simulink model "cic_filter_test_newnew_dec2_nonpoly_3"  (Simulink 7.4)
settings: Solver=ode45  StartTime=0.0  StopTime=50000  RelTol=1e-3
libraries: xbsIndex_r4 x203, simulink x3, xrbsComm_r4 x1, xps_library x1
(part 2 of 2)

== system cic_filter_test_newnew_dec2_nonpoly_3/CIC Filter/Integrator3 ==
  In1 : Inport  OutDataType=sfix(16)  OutScaling=2^0
  Accumulator : xbsIndex_r4/Accumulator  operation=Add  n_bits=output_bitwidth  overflow=Wrap  scale=1  rst=off  hasbypass=off  en=off  dbl_ovrd=off  use_behavioral_HDL=on  implementation=Fabric  block_type=accum
      settings: infoedit="Adder or subtractor-based accumulator.   Output type and binary point position match the input.<P><P>Hardware notes: When \"Reinitialize with Input 'b' on Reset\" is selected, the accumulator is forced to run at the system rate even if the input 'b' is running at a slower rate."  xl_area=[53 106 0 106 0 0 0]  block_version=VER_STRING_GOES_HERE
  Out1 : Outport  OutDataType=sfix(16)  OutScaling=2^0
  wires:
  Accumulator/1 -> Out1/1
  In1/1 -> Accumulator/1

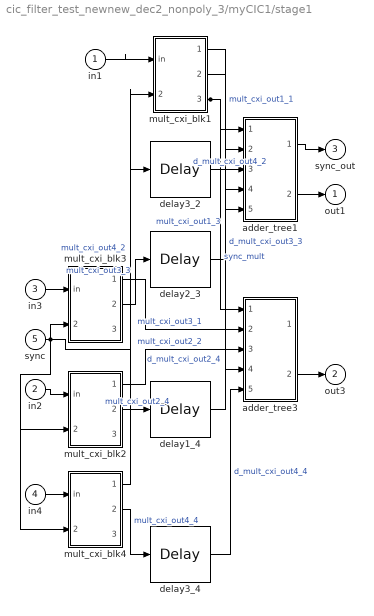
== system cic_filter_test_newnew_dec2_nonpoly_3/myCIC1/stage1 ==
  in1 : Inport
  in2 : Inport  Port=2
  in3 : Inport  Port=3
  in4 : Inport  Port=4
  sync : Inport  Port=5
  adder_tree1 : Subsystem
  adder_tree3 : Subsystem
  delay1_4 : xbsIndex_r4/Delay  en=off  latency=1  dbl_ovrd=off  reg_retiming=off  block_type=delay
      settings: block_version=11.4
  delay2_3 : xbsIndex_r4/Delay  en=off  latency=1  dbl_ovrd=off  reg_retiming=off  block_type=delay
      settings: block_version=11.4
  delay3_2 : xbsIndex_r4/Delay  en=off  latency=1  dbl_ovrd=off  reg_retiming=off  block_type=delay
      settings: block_version=11.4
  delay3_4 : xbsIndex_r4/Delay  en=off  latency=1  dbl_ovrd=off  reg_retiming=off  block_type=delay
      settings: block_version=11.4
  mult_cxi_blk1 : Subsystem
  mult_cxi_blk2 : Subsystem
  mult_cxi_blk3 : Subsystem
  mult_cxi_blk4 : Subsystem
  out1 : Outport
  out3 : Outport  Port=2
  sync_out : Outport  Port=3
  wires:
  sync/1 -> mult_cxi_blk4/2(sync), mult_cxi_blk2/2(sync), mult_cxi_blk1/2(sync), mult_cxi_blk3/2(sync)
  mult_cxi_blk1/3(sync_out) -> adder_tree3/1(sync), adder_tree1/1(sync)  "sync_mult"
  delay3_4/1 -> adder_tree3/5(din_4)  "d_mult_cxi_out4_4"
  mult_cxi_blk2/1(out1) -> adder_tree3/3(din_2)  "mult_cxi_out2_2"
  adder_tree1/2(dout) -> out1/1
  delay1_4/1 -> adder_tree1/5(din_4)  "d_mult_cxi_out2_4"
  delay3_2/1 -> adder_tree1/3(din_2)  "d_mult_cxi_out4_2"
  mult_cxi_blk4/2(out2) -> delay3_4/1  "mult_cxi_out4_4"
  mult_cxi_blk4/1(out1) -> delay3_2/1  "mult_cxi_out4_2"
  mult_cxi_blk3/2(out2) -> delay2_3/1  "mult_cxi_out3_3"
  mult_cxi_blk2/2(out2) -> delay1_4/1  "mult_cxi_out2_4"
  in3/1 -> mult_cxi_blk3/1(in)
  in1/1 -> mult_cxi_blk1/1(in)
  in2/1 -> mult_cxi_blk2/1(in)
  in4/1 -> mult_cxi_blk4/1(in)
  mult_cxi_blk1/1(out1) -> adder_tree1/2(din_1)  "mult_cxi_out1_1"
  delay2_3/1 -> adder_tree1/4(din_3)  "d_mult_cxi_out3_3"
  adder_tree1/1(sync_out) -> sync_out/1
  mult_cxi_blk3/1(out1) -> adder_tree3/2(din_1)  "mult_cxi_out3_1"
  mult_cxi_blk1/2(out2) -> adder_tree3/4(din_3)  "mult_cxi_out1_3"
  adder_tree3/2(dout) -> out3/1

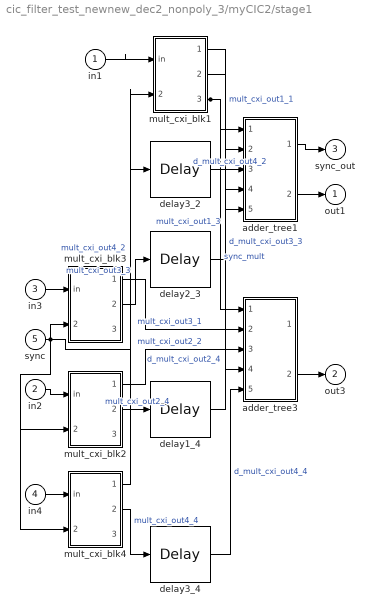
== system cic_filter_test_newnew_dec2_nonpoly_3/myCIC2/stage1 ==
  in1 : Inport
  in2 : Inport  Port=2
  in3 : Inport  Port=3
  in4 : Inport  Port=4
  sync : Inport  Port=5
  adder_tree1 : Subsystem
  adder_tree3 : Subsystem
  delay1_4 : xbsIndex_r4/Delay  en=off  latency=1  dbl_ovrd=off  reg_retiming=off  block_type=delay
      settings: block_version=11.4
  delay2_3 : xbsIndex_r4/Delay  en=off  latency=1  dbl_ovrd=off  reg_retiming=off  block_type=delay
      settings: block_version=11.4
  delay3_2 : xbsIndex_r4/Delay  en=off  latency=1  dbl_ovrd=off  reg_retiming=off  block_type=delay
      settings: block_version=11.4
  delay3_4 : xbsIndex_r4/Delay  en=off  latency=1  dbl_ovrd=off  reg_retiming=off  block_type=delay
      settings: block_version=11.4
  mult_cxi_blk1 : Subsystem
  mult_cxi_blk2 : Subsystem
  mult_cxi_blk3 : Subsystem
  mult_cxi_blk4 : Subsystem
  out1 : Outport
  out3 : Outport  Port=2
  sync_out : Outport  Port=3
  wires:
  sync/1 -> mult_cxi_blk4/2(sync), mult_cxi_blk2/2(sync), mult_cxi_blk1/2(sync), mult_cxi_blk3/2(sync)
  mult_cxi_blk1/3(sync_out) -> adder_tree3/1(sync), adder_tree1/1(sync)  "sync_mult"
  delay3_4/1 -> adder_tree3/5(din_4)  "d_mult_cxi_out4_4"
  mult_cxi_blk2/1(out1) -> adder_tree3/3(din_2)  "mult_cxi_out2_2"
  adder_tree1/2(dout) -> out1/1
  delay1_4/1 -> adder_tree1/5(din_4)  "d_mult_cxi_out2_4"
  delay3_2/1 -> adder_tree1/3(din_2)  "d_mult_cxi_out4_2"
  mult_cxi_blk4/2(out2) -> delay3_4/1  "mult_cxi_out4_4"
  mult_cxi_blk4/1(out1) -> delay3_2/1  "mult_cxi_out4_2"
  mult_cxi_blk3/2(out2) -> delay2_3/1  "mult_cxi_out3_3"
  mult_cxi_blk2/2(out2) -> delay1_4/1  "mult_cxi_out2_4"
  in3/1 -> mult_cxi_blk3/1(in)
  in1/1 -> mult_cxi_blk1/1(in)
  in2/1 -> mult_cxi_blk2/1(in)
  in4/1 -> mult_cxi_blk4/1(in)
  mult_cxi_blk1/1(out1) -> adder_tree1/2(din_1)  "mult_cxi_out1_1"
  delay2_3/1 -> adder_tree1/4(din_3)  "d_mult_cxi_out3_3"
  adder_tree1/1(sync_out) -> sync_out/1
  mult_cxi_blk3/1(out1) -> adder_tree3/2(din_1)  "mult_cxi_out3_1"
  mult_cxi_blk1/2(out2) -> adder_tree3/4(din_3)  "mult_cxi_out1_3"
  adder_tree3/2(dout) -> out3/1

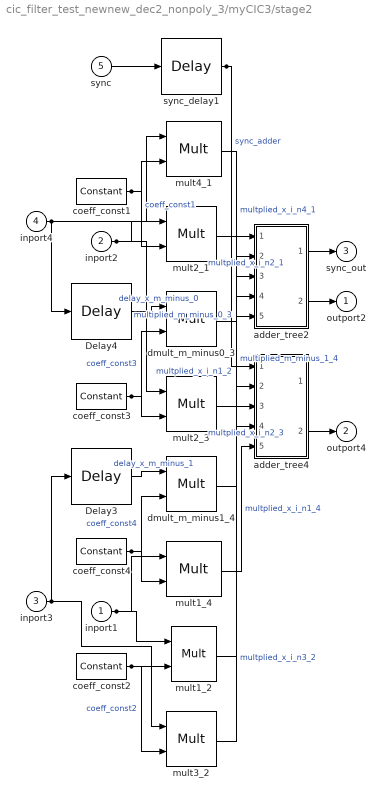
== system cic_filter_test_newnew_dec2_nonpoly_3/myCIC3/stage2 ==
  inport1 : Inport
  inport2 : Inport  Port=2
  inport3 : Inport  Port=3
  inport4 : Inport  Port=4
  sync : Inport  Port=5
  Delay3 : xbsIndex_r4/Delay  en=off  latency=1  dbl_ovrd=off  reg_retiming=off  block_type=delay
      settings: block_version=11.4
  Delay4 : xbsIndex_r4/Delay  en=off  latency=1  dbl_ovrd=off  reg_retiming=off  block_type=delay
      settings: block_version=11.4
  adder_tree2 : Subsystem
  adder_tree4 : Subsystem
  coeff_const1 : xbsIndex_r4/Constant  arith_type=Unsigned  const=1  n_bits=3  bin_pt=0  explicit_period=off  period=1  equ=P=C  opselect=C  inp2=PCIN>>17  opr=+  inp1=P  carry=CIN  dbl_ovrd=off  block_type=constant
      settings: block_version=11.4
  coeff_const2 : xbsIndex_r4/Constant  arith_type=Unsigned  const=3  n_bits=3  bin_pt=0  explicit_period=off  period=1  equ=P=C  opselect=C  inp2=PCIN>>17  opr=+  inp1=P  carry=CIN  dbl_ovrd=off  block_type=constant
      settings: block_version=11.4
  coeff_const3 : xbsIndex_r4/Constant  arith_type=Unsigned  const=3  n_bits=3  bin_pt=0  explicit_period=off  period=1  equ=P=C  opselect=C  inp2=PCIN>>17  opr=+  inp1=P  carry=CIN  dbl_ovrd=off  block_type=constant
      settings: block_version=11.4
  coeff_const4 : xbsIndex_r4/Constant  arith_type=Unsigned  const=1  n_bits=3  bin_pt=0  explicit_period=off  period=1  equ=P=C  opselect=C  inp2=PCIN>>17  opr=+  inp1=P  carry=CIN  dbl_ovrd=off  block_type=constant
      settings: block_version=11.4
  dmult_m_minus0_3 : xbsIndex_r4/Mult  precision=Full  arith_type="Signed  (2's comp)"  n_bits=16  bin_pt=14  quantization=Truncate  overflow=Wrap  en=off  latency=2  dbl_ovrd=off  use_behavioral_HDL=off  opt=Speed  use_embedded=on  optimum_pipeline=off  pipeline=on  use_rpm=on  placement_style=Triangular  block_type=mult
      settings: block_version=11.4
  dmult_m_minus1_4 : xbsIndex_r4/Mult  precision=Full  arith_type="Signed  (2's comp)"  n_bits=16  bin_pt=14  quantization=Truncate  overflow=Wrap  en=off  latency=2  dbl_ovrd=off  use_behavioral_HDL=off  opt=Speed  use_embedded=on  optimum_pipeline=off  pipeline=on  use_rpm=on  placement_style=Triangular  block_type=mult
      settings: block_version=11.4
  mult1_2 : xbsIndex_r4/Mult  precision=Full  arith_type="Signed  (2's comp)"  n_bits=16  bin_pt=14  quantization=Truncate  overflow=Wrap  en=off  latency=2  dbl_ovrd=off  use_behavioral_HDL=off  opt=Speed  use_embedded=on  optimum_pipeline=off  pipeline=on  use_rpm=on  placement_style=Triangular  block_type=mult
      settings: block_version=11.4
  mult1_4 : xbsIndex_r4/Mult  precision=Full  arith_type="Signed  (2's comp)"  n_bits=16  bin_pt=14  quantization=Truncate  overflow=Wrap  en=off  latency=2  dbl_ovrd=off  use_behavioral_HDL=off  opt=Speed  use_embedded=on  optimum_pipeline=off  pipeline=on  use_rpm=on  placement_style=Triangular  block_type=mult
      settings: block_version=11.4
  mult2_1 : xbsIndex_r4/Mult  precision=Full  arith_type="Signed  (2's comp)"  n_bits=16  bin_pt=14  quantization=Truncate  overflow=Wrap  en=off  latency=2  dbl_ovrd=off  use_behavioral_HDL=off  opt=Speed  use_embedded=on  optimum_pipeline=off  pipeline=on  use_rpm=on  placement_style=Triangular  block_type=mult
      settings: block_version=11.4
  mult2_3 : xbsIndex_r4/Mult  precision=Full  arith_type="Signed  (2's comp)"  n_bits=16  bin_pt=14  quantization=Truncate  overflow=Wrap  en=off  latency=2  dbl_ovrd=off  use_behavioral_HDL=off  opt=Speed  use_embedded=on  optimum_pipeline=off  pipeline=on  use_rpm=on  placement_style=Triangular  block_type=mult
      settings: block_version=11.4
  mult3_2 : xbsIndex_r4/Mult  precision=Full  arith_type="Signed  (2's comp)"  n_bits=16  bin_pt=14  quantization=Truncate  overflow=Wrap  en=off  latency=2  dbl_ovrd=off  use_behavioral_HDL=off  opt=Speed  use_embedded=on  optimum_pipeline=off  pipeline=on  use_rpm=on  placement_style=Triangular  block_type=mult
      settings: block_version=11.4
  mult4_1 : xbsIndex_r4/Mult  precision=Full  arith_type="Signed  (2's comp)"  n_bits=16  bin_pt=14  quantization=Truncate  overflow=Wrap  en=off  latency=2  dbl_ovrd=off  use_behavioral_HDL=off  opt=Speed  use_embedded=on  optimum_pipeline=off  pipeline=on  use_rpm=on  placement_style=Triangular  block_type=mult
      settings: block_version=11.4
  sync_delay1 : xbsIndex_r4/Delay  en=off  latency=2  dbl_ovrd=off  reg_retiming=off  block_type=delay
      settings: block_version=11.4
  outport2 : Outport
  outport4 : Outport  Port=2
  sync_out : Outport  Port=3
  wires:
  inport1/1 -> mult1_2/1, mult1_4/1
  coeff_const4/1 -> mult1_4/2, dmult_m_minus1_4/2  "coeff_const4"
  inport2/1 -> mult2_1/1, mult2_3/1
  coeff_const3/1 -> mult2_3/2, dmult_m_minus0_3/2  "coeff_const3"
  inport3/1 -> mult3_2/1, Delay3/1
  coeff_const2/1 -> mult1_2/2, mult3_2/2  "coeff_const2"
  inport4/1 -> Delay4/1, mult4_1/1
  coeff_const1/1 -> mult4_1/2, mult2_1/2  "coeff_const1"
  sync_delay1/1 -> adder_tree4/1(sync), adder_tree2/1(sync)  "sync_adder"
  mult1_4/1 -> adder_tree4/5(din_4)  "multplied_x_i_n1_4"
  mult3_2/1 -> adder_tree4/3(din_2)  "multplied_x_i_n3_2"
  adder_tree2/2(dout) -> outport2/1
  dmult_m_minus1_4/1 -> adder_tree2/5(din_4)  "multiplied_m_minus_1_4"
  mult1_2/1 -> adder_tree2/3(din_2)  "multplied_x_i_n1_2"
  sync/1 -> sync_delay1/1
  Delay4/1 -> dmult_m_minus0_3/1  "delay_x_m_minus_0"
  Delay3/1 -> dmult_m_minus1_4/1  "delay_x_m_minus_1"
  mult2_1/1 -> adder_tree2/2(din_1)  "multplied_x_i_n2_1"
  dmult_m_minus0_3/1 -> adder_tree2/4(din_3)  "multiplied_m_minus_0_3"
  adder_tree2/1(sync_out) -> sync_out/1
  mult4_1/1 -> adder_tree4/2(din_1)  "multplied_x_i_n4_1"
  mult2_3/1 -> adder_tree4/4(din_3)  "multplied_x_i_n2_3"
  adder_tree4/2(dout) -> outport4/1

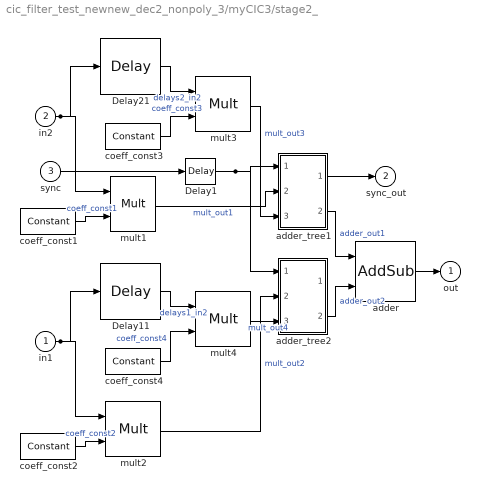
== system cic_filter_test_newnew_dec2_nonpoly_3/myCIC3/stage2_ ==
  in1 : Inport
  in2 : Inport  Port=2
  sync : Inport  Port=3
  Delay1 : xbsIndex_r4/Delay  en=off  latency=2  dbl_ovrd=off  reg_retiming=off  block_type=delay
      settings: block_version=11.4
  Delay11 : xbsIndex_r4/Delay  en=off  latency=1  dbl_ovrd=off  reg_retiming=off  block_type=delay
      settings: block_version=11.4
  Delay21 : xbsIndex_r4/Delay  en=off  latency=1  dbl_ovrd=off  reg_retiming=off  block_type=delay
      settings: block_version=11.4
  adder : xbsIndex_r4/AddSub  mode=Addition  use_carryin=off  use_carryout=off  en=off  latency=1  precision=Full  arith_type=Unsigned  n_bits=16  bin_pt=14  quantization=Truncate  overflow=Wrap  dbl_ovrd=off  use_behavioral_HDL=off  hw_selection=Fabric  pipelined=off  block_type=addsub
  adder_tree1 : Subsystem
  adder_tree2 : Subsystem
  coeff_const1 : xbsIndex_r4/Constant  arith_type=Unsigned  const=1  n_bits=3  bin_pt=0  explicit_period=off  period=1  equ=P=C  opselect=C  inp2=PCIN>>17  opr=+  inp1=P  carry=CIN  dbl_ovrd=off  block_type=constant
      settings: block_version=11.4
  coeff_const2 : xbsIndex_r4/Constant  arith_type=Unsigned  const=3  n_bits=3  bin_pt=0  explicit_period=off  period=1  equ=P=C  opselect=C  inp2=PCIN>>17  opr=+  inp1=P  carry=CIN  dbl_ovrd=off  block_type=constant
      settings: block_version=11.4
  coeff_const3 : xbsIndex_r4/Constant  arith_type=Unsigned  const=3  n_bits=3  bin_pt=0  explicit_period=off  period=1  equ=P=C  opselect=C  inp2=PCIN>>17  opr=+  inp1=P  carry=CIN  dbl_ovrd=off  block_type=constant
      settings: block_version=11.4
  coeff_const4 : xbsIndex_r4/Constant  arith_type=Unsigned  const=1  n_bits=3  bin_pt=0  explicit_period=off  period=1  equ=P=C  opselect=C  inp2=PCIN>>17  opr=+  inp1=P  carry=CIN  dbl_ovrd=off  block_type=constant
      settings: block_version=11.4
  mult{1..4} (4 alike) : xbsIndex_r4/Mult  precision=Full  arith_type="Signed  (2's comp)"  n_bits=16  bin_pt=14  quantization=Truncate  overflow=Wrap  en=off  latency=2  dbl_ovrd=off  use_behavioral_HDL=off  opt=Speed  use_embedded=on  optimum_pipeline=off  pipeline=on  use_rpm=on  placement_style=Triangular  block_type=mult
      settings: block_version=11.4
  out : Outport
  sync_out : Outport  Port=2
  wires:
  in2/1 -> mult1/1, Delay21/1
  in1/1 -> Delay11/1, mult2/1
  sync/1 -> Delay1/1
  adder_tree2/2(dout) -> adder/2  "adder_out2"
  mult2/1 -> adder_tree2/2(din_1)  "mult_out2"
  mult3/1 -> adder_tree1/3(din_2)  "mult_out3"
  coeff_const4/1 -> mult4/2  "coeff_const4"
  Delay21/1 -> mult3/1  "delays2_in2"
  coeff_const2/1 -> mult2/2  "coeff_const2"
  coeff_const1/1 -> mult1/2  "coeff_const1"
  coeff_const3/1 -> mult3/2  "coeff_const3"
  Delay11/1 -> mult4/1  "delays1_in2"
  mult1/1 -> adder_tree1/2(din_1)  "mult_out1"
  adder_tree1/1(sync_out) -> sync_out/1
  mult4/1 -> adder_tree2/3(din_2)  "mult_out4"
  adder_tree1/2(dout) -> adder/1  "adder_out1"
  adder/1 -> out/1
  Delay1/1 -> adder_tree1/1(sync), adder_tree2/1(sync)

== system cic_filter_test_newnew_dec2_nonpoly_3/npcic nonpoly/stage1 ==
  in : Inport
  sync : Inport  Port=2
  Down_sample0 : xbsIndex_r4/Down Sample  sample_ratio=2  sample_phase="Last Value of Frame  (most efficient)"  en=off  latency=1  dbl_ovrd=off  block_type=dsamp
      settings: block_version=11.4
  polynomial : Subsystem
  out : Outport
  sync_out : Outport  Port=2
  wires:
  polynomial/1(out) -> Down_sample0/1  "poly_out"
  polynomial/2(sync_out) -> sync_out/1
  in/1 -> polynomial/1(in)
  sync/1 -> polynomial/2(sync)
  Down_sample0/1 -> out/1

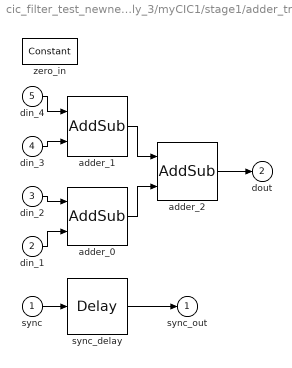
== system cic_filter_test_newnew_dec2_nonpoly_3/myCIC1/stage1/adder_tree1 ==
  sync : Inport
  din_1 : Inport  Port=2
  din_2 : Inport  Port=3
  din_3 : Inport  Port=4
  din_4 : Inport  Port=5
  adder_0 : xbsIndex_r4/AddSub  mode=Addition  use_carryin=off  use_carryout=off  en=off  latency=1  precision=Full  arith_type=Unsigned  n_bits=16  bin_pt=14  quantization="Round  (unbiased: +/- Inf)"  overflow=Saturate  dbl_ovrd=off  use_behavioral_HDL=on  hw_selection=Fabric  pipelined=off  block_type=addsub
  adder_1 : xbsIndex_r4/AddSub  mode=Addition  use_carryin=off  use_carryout=off  en=off  latency=1  precision=Full  arith_type=Unsigned  n_bits=16  bin_pt=14  quantization="Round  (unbiased: +/- Inf)"  overflow=Saturate  dbl_ovrd=off  use_behavioral_HDL=on  hw_selection=Fabric  pipelined=off  block_type=addsub
  adder_2 : xbsIndex_r4/AddSub  mode=Addition  use_carryin=off  use_carryout=off  en=off  latency=1  precision=Full  arith_type=Unsigned  n_bits=16  bin_pt=14  quantization="Round  (unbiased: +/- Inf)"  overflow=Saturate  dbl_ovrd=off  use_behavioral_HDL=on  hw_selection=Fabric  pipelined=off  block_type=addsub
  sync_delay : xbsIndex_r4/Delay  en=off  latency=2  dbl_ovrd=off  reg_retiming=off  block_type=delay
      settings: block_version=11.4
  zero_in : xbsIndex_r4/Constant  arith_type=Unsigned  const=0  n_bits=18  bin_pt=17  explicit_period=off  period=1  equ=P=C  opselect=C  inp2=PCIN>>17  opr=+  inp1=P  carry=CIN  dbl_ovrd=off  block_type=constant
      settings: block_version=11.4
  sync_out : Outport
  dout : Outport  Port=2
  wires:
  adder_0/1 -> adder_2/2
  din_4/1 -> adder_1/1
  din_1/1 -> adder_0/2
  sync_delay/1 -> sync_out/1
  sync/1 -> sync_delay/1
  din_2/1 -> adder_0/1
  din_3/1 -> adder_1/2
  adder_1/1 -> adder_2/1
  adder_2/1 -> dout/1

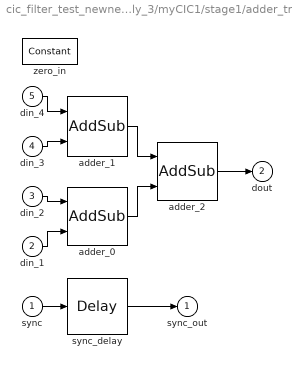
== system cic_filter_test_newnew_dec2_nonpoly_3/myCIC1/stage1/adder_tree3 ==
  sync : Inport
  din_1 : Inport  Port=2
  din_2 : Inport  Port=3
  din_3 : Inport  Port=4
  din_4 : Inport  Port=5
  adder_0 : xbsIndex_r4/AddSub  mode=Addition  use_carryin=off  use_carryout=off  en=off  latency=1  precision=Full  arith_type=Unsigned  n_bits=16  bin_pt=14  quantization="Round  (unbiased: +/- Inf)"  overflow=Saturate  dbl_ovrd=off  use_behavioral_HDL=on  hw_selection=Fabric  pipelined=off  block_type=addsub
  adder_1 : xbsIndex_r4/AddSub  mode=Addition  use_carryin=off  use_carryout=off  en=off  latency=1  precision=Full  arith_type=Unsigned  n_bits=16  bin_pt=14  quantization="Round  (unbiased: +/- Inf)"  overflow=Saturate  dbl_ovrd=off  use_behavioral_HDL=on  hw_selection=Fabric  pipelined=off  block_type=addsub
  adder_2 : xbsIndex_r4/AddSub  mode=Addition  use_carryin=off  use_carryout=off  en=off  latency=1  precision=Full  arith_type=Unsigned  n_bits=16  bin_pt=14  quantization="Round  (unbiased: +/- Inf)"  overflow=Saturate  dbl_ovrd=off  use_behavioral_HDL=on  hw_selection=Fabric  pipelined=off  block_type=addsub
  sync_delay : xbsIndex_r4/Delay  en=off  latency=2  dbl_ovrd=off  reg_retiming=off  block_type=delay
      settings: block_version=11.4
  zero_in : xbsIndex_r4/Constant  arith_type=Unsigned  const=0  n_bits=18  bin_pt=17  explicit_period=off  period=1  equ=P=C  opselect=C  inp2=PCIN>>17  opr=+  inp1=P  carry=CIN  dbl_ovrd=off  block_type=constant
      settings: block_version=11.4
  sync_out : Outport
  dout : Outport  Port=2
  wires:
  adder_0/1 -> adder_2/2
  din_4/1 -> adder_1/1
  din_1/1 -> adder_0/2
  sync_delay/1 -> sync_out/1
  sync/1 -> sync_delay/1
  din_2/1 -> adder_0/1
  din_3/1 -> adder_1/2
  adder_1/1 -> adder_2/1
  adder_2/1 -> dout/1

== system cic_filter_test_newnew_dec2_nonpoly_3/myCIC1/stage1/mult_cxi_blk1 ==
  in : Inport
  sync : Inport  Port=2
  adder_tree2 : Subsystem
  delay1 : xbsIndex_r4/Delay  en=off  latency=1  dbl_ovrd=off  reg_retiming=off  block_type=delay
      settings: block_version=11.4
  shift2 : xbsIndex_r4/Shift  shift_dir=Left  shift_bits=1  en=off  latency=0  precision=Full  arith_type="Signed  (2's comp)"  n_bits=16  bin_pt=14  quantization=Truncate  overflow=Wrap  dbl_ovrd=off  block_type=shift
  sync_delay : xbsIndex_r4/Delay  en=off  latency=1  dbl_ovrd=off  reg_retiming=off  block_type=delay
      settings: block_version=11.4
  out1 : Outport
  out2 : Outport  Port=2
  sync_out : Outport  Port=3
  wires:
  in/1 -> delay1/1, adder_tree2/1(sync), shift2/1, adder_tree2/2(din_1)  "adder_trees_out1"
  sync/1 -> sync_delay/1
  delay1/1 -> out1/1  "out1"
  shift2/1 -> adder_tree2/3(din_2)  "shift_out2"
  adder_tree2/2(dout) -> out2/1  "out2"
  sync_delay/1 -> sync_out/1

== system cic_filter_test_newnew_dec2_nonpoly_3/myCIC1/stage1/mult_cxi_blk2 ==
  in : Inport
  sync : Inport  Port=2
  adder_tree1 : Subsystem
  delay2 : xbsIndex_r4/Delay  en=off  latency=1  dbl_ovrd=off  reg_retiming=off  block_type=delay
      settings: block_version=11.4
  shift2 : xbsIndex_r4/Shift  shift_dir=Left  shift_bits=1  en=off  latency=0  precision=Full  arith_type="Signed  (2's comp)"  n_bits=16  bin_pt=14  quantization=Truncate  overflow=Wrap  dbl_ovrd=off  block_type=shift
  sync_delay : xbsIndex_r4/Delay  en=off  latency=1  dbl_ovrd=off  reg_retiming=off  block_type=delay
      settings: block_version=11.4
  out1 : Outport
  out2 : Outport  Port=2
  sync_out : Outport  Port=3
  wires:
  in/1 -> delay2/1, adder_tree1/1(sync), shift2/1, adder_tree1/2(din_1)  "adder_trees_out2"
  sync/1 -> sync_delay/1
  adder_tree1/2(dout) -> out1/1  "out1"
  shift2/1 -> adder_tree1/3(din_2)  "shift_out2"
  delay2/1 -> out2/1  "out2"
  sync_delay/1 -> sync_out/1

== system cic_filter_test_newnew_dec2_nonpoly_3/myCIC1/stage1/mult_cxi_blk3 ==
  in : Inport
  sync : Inport  Port=2
  adder_tree2 : Subsystem
  delay1 : xbsIndex_r4/Delay  en=off  latency=1  dbl_ovrd=off  reg_retiming=off  block_type=delay
      settings: block_version=11.4
  shift2 : xbsIndex_r4/Shift  shift_dir=Left  shift_bits=1  en=off  latency=0  precision=Full  arith_type="Signed  (2's comp)"  n_bits=16  bin_pt=14  quantization=Truncate  overflow=Wrap  dbl_ovrd=off  block_type=shift
  sync_delay : xbsIndex_r4/Delay  en=off  latency=1  dbl_ovrd=off  reg_retiming=off  block_type=delay
      settings: block_version=11.4
  out1 : Outport
  out2 : Outport  Port=2
  sync_out : Outport  Port=3
  wires:
  in/1 -> delay1/1, adder_tree2/1(sync), shift2/1, adder_tree2/2(din_1)  "adder_trees_out1"
  sync/1 -> sync_delay/1
  delay1/1 -> out1/1  "out1"
  shift2/1 -> adder_tree2/3(din_2)  "shift_out2"
  adder_tree2/2(dout) -> out2/1  "out2"
  sync_delay/1 -> sync_out/1

== system cic_filter_test_newnew_dec2_nonpoly_3/myCIC1/stage1/mult_cxi_blk4 ==
  in : Inport
  sync : Inport  Port=2
  adder_tree1 : Subsystem
  delay2 : xbsIndex_r4/Delay  en=off  latency=1  dbl_ovrd=off  reg_retiming=off  block_type=delay
      settings: block_version=11.4
  shift2 : xbsIndex_r4/Shift  shift_dir=Left  shift_bits=1  en=off  latency=0  precision=Full  arith_type="Signed  (2's comp)"  n_bits=16  bin_pt=14  quantization=Truncate  overflow=Wrap  dbl_ovrd=off  block_type=shift
  sync_delay : xbsIndex_r4/Delay  en=off  latency=1  dbl_ovrd=off  reg_retiming=off  block_type=delay
      settings: block_version=11.4
  out1 : Outport
  out2 : Outport  Port=2
  sync_out : Outport  Port=3
  wires:
  in/1 -> delay2/1, adder_tree1/1(sync), shift2/1, adder_tree1/2(din_1)  "adder_trees_out2"
  sync/1 -> sync_delay/1
  adder_tree1/2(dout) -> out1/1  "out1"
  shift2/1 -> adder_tree1/3(din_2)  "shift_out2"
  delay2/1 -> out2/1  "out2"
  sync_delay/1 -> sync_out/1

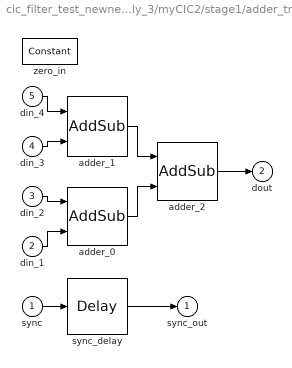
== system cic_filter_test_newnew_dec2_nonpoly_3/myCIC2/stage1/adder_tree1 ==
  sync : Inport
  din_1 : Inport  Port=2
  din_2 : Inport  Port=3
  din_3 : Inport  Port=4
  din_4 : Inport  Port=5
  adder_0 : xbsIndex_r4/AddSub  mode=Addition  use_carryin=off  use_carryout=off  en=off  latency=1  precision=Full  arith_type=Unsigned  n_bits=16  bin_pt=14  quantization="Round  (unbiased: +/- Inf)"  overflow=Saturate  dbl_ovrd=off  use_behavioral_HDL=on  hw_selection=Fabric  pipelined=off  block_type=addsub
  adder_1 : xbsIndex_r4/AddSub  mode=Addition  use_carryin=off  use_carryout=off  en=off  latency=1  precision=Full  arith_type=Unsigned  n_bits=16  bin_pt=14  quantization="Round  (unbiased: +/- Inf)"  overflow=Saturate  dbl_ovrd=off  use_behavioral_HDL=on  hw_selection=Fabric  pipelined=off  block_type=addsub
  adder_2 : xbsIndex_r4/AddSub  mode=Addition  use_carryin=off  use_carryout=off  en=off  latency=1  precision=Full  arith_type=Unsigned  n_bits=16  bin_pt=14  quantization="Round  (unbiased: +/- Inf)"  overflow=Saturate  dbl_ovrd=off  use_behavioral_HDL=on  hw_selection=Fabric  pipelined=off  block_type=addsub
  sync_delay : xbsIndex_r4/Delay  en=off  latency=2  dbl_ovrd=off  reg_retiming=off  block_type=delay
      settings: block_version=11.4
  zero_in : xbsIndex_r4/Constant  arith_type=Unsigned  const=0  n_bits=18  bin_pt=17  explicit_period=off  period=1  equ=P=C  opselect=C  inp2=PCIN>>17  opr=+  inp1=P  carry=CIN  dbl_ovrd=off  block_type=constant
      settings: block_version=11.4
  sync_out : Outport
  dout : Outport  Port=2
  wires:
  adder_0/1 -> adder_2/2
  din_4/1 -> adder_1/1
  din_1/1 -> adder_0/2
  sync_delay/1 -> sync_out/1
  sync/1 -> sync_delay/1
  din_2/1 -> adder_0/1
  din_3/1 -> adder_1/2
  adder_1/1 -> adder_2/1
  adder_2/1 -> dout/1

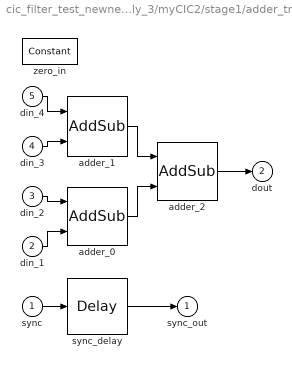
== system cic_filter_test_newnew_dec2_nonpoly_3/myCIC2/stage1/adder_tree3 ==
  sync : Inport
  din_1 : Inport  Port=2
  din_2 : Inport  Port=3
  din_3 : Inport  Port=4
  din_4 : Inport  Port=5
  adder_0 : xbsIndex_r4/AddSub  mode=Addition  use_carryin=off  use_carryout=off  en=off  latency=1  precision=Full  arith_type=Unsigned  n_bits=16  bin_pt=14  quantization="Round  (unbiased: +/- Inf)"  overflow=Saturate  dbl_ovrd=off  use_behavioral_HDL=on  hw_selection=Fabric  pipelined=off  block_type=addsub
  adder_1 : xbsIndex_r4/AddSub  mode=Addition  use_carryin=off  use_carryout=off  en=off  latency=1  precision=Full  arith_type=Unsigned  n_bits=16  bin_pt=14  quantization="Round  (unbiased: +/- Inf)"  overflow=Saturate  dbl_ovrd=off  use_behavioral_HDL=on  hw_selection=Fabric  pipelined=off  block_type=addsub
  adder_2 : xbsIndex_r4/AddSub  mode=Addition  use_carryin=off  use_carryout=off  en=off  latency=1  precision=Full  arith_type=Unsigned  n_bits=16  bin_pt=14  quantization="Round  (unbiased: +/- Inf)"  overflow=Saturate  dbl_ovrd=off  use_behavioral_HDL=on  hw_selection=Fabric  pipelined=off  block_type=addsub
  sync_delay : xbsIndex_r4/Delay  en=off  latency=2  dbl_ovrd=off  reg_retiming=off  block_type=delay
      settings: block_version=11.4
  zero_in : xbsIndex_r4/Constant  arith_type=Unsigned  const=0  n_bits=18  bin_pt=17  explicit_period=off  period=1  equ=P=C  opselect=C  inp2=PCIN>>17  opr=+  inp1=P  carry=CIN  dbl_ovrd=off  block_type=constant
      settings: block_version=11.4
  sync_out : Outport
  dout : Outport  Port=2
  wires:
  adder_0/1 -> adder_2/2
  din_4/1 -> adder_1/1
  din_1/1 -> adder_0/2
  sync_delay/1 -> sync_out/1
  sync/1 -> sync_delay/1
  din_2/1 -> adder_0/1
  din_3/1 -> adder_1/2
  adder_1/1 -> adder_2/1
  adder_2/1 -> dout/1

== system cic_filter_test_newnew_dec2_nonpoly_3/myCIC2/stage1/mult_cxi_blk1 ==
  in : Inport
  sync : Inport  Port=2
  adder_tree2 : Subsystem
  delay1 : xbsIndex_r4/Delay  en=off  latency=1  dbl_ovrd=off  reg_retiming=off  block_type=delay
      settings: block_version=11.4
  shift2 : xbsIndex_r4/Shift  shift_dir=Left  shift_bits=1  en=off  latency=0  precision=Full  arith_type="Signed  (2's comp)"  n_bits=16  bin_pt=14  quantization=Truncate  overflow=Wrap  dbl_ovrd=off  block_type=shift
  sync_delay : xbsIndex_r4/Delay  en=off  latency=1  dbl_ovrd=off  reg_retiming=off  block_type=delay
      settings: block_version=11.4
  out1 : Outport
  out2 : Outport  Port=2
  sync_out : Outport  Port=3
  wires:
  in/1 -> delay1/1, adder_tree2/1(sync), shift2/1, adder_tree2/2(din_1)  "adder_trees_out1"
  sync/1 -> sync_delay/1
  delay1/1 -> out1/1  "out1"
  shift2/1 -> adder_tree2/3(din_2)  "shift_out2"
  adder_tree2/2(dout) -> out2/1  "out2"
  sync_delay/1 -> sync_out/1

== system cic_filter_test_newnew_dec2_nonpoly_3/myCIC2/stage1/mult_cxi_blk2 ==
  in : Inport
  sync : Inport  Port=2
  adder_tree1 : Subsystem
  delay2 : xbsIndex_r4/Delay  en=off  latency=1  dbl_ovrd=off  reg_retiming=off  block_type=delay
      settings: block_version=11.4
  shift2 : xbsIndex_r4/Shift  shift_dir=Left  shift_bits=1  en=off  latency=0  precision=Full  arith_type="Signed  (2's comp)"  n_bits=16  bin_pt=14  quantization=Truncate  overflow=Wrap  dbl_ovrd=off  block_type=shift
  sync_delay : xbsIndex_r4/Delay  en=off  latency=1  dbl_ovrd=off  reg_retiming=off  block_type=delay
      settings: block_version=11.4
  out1 : Outport
  out2 : Outport  Port=2
  sync_out : Outport  Port=3
  wires:
  in/1 -> delay2/1, adder_tree1/1(sync), shift2/1, adder_tree1/2(din_1)  "adder_trees_out2"
  sync/1 -> sync_delay/1
  adder_tree1/2(dout) -> out1/1  "out1"
  shift2/1 -> adder_tree1/3(din_2)  "shift_out2"
  delay2/1 -> out2/1  "out2"
  sync_delay/1 -> sync_out/1

== system cic_filter_test_newnew_dec2_nonpoly_3/myCIC2/stage1/mult_cxi_blk3 ==
  in : Inport
  sync : Inport  Port=2
  adder_tree2 : Subsystem
  delay1 : xbsIndex_r4/Delay  en=off  latency=1  dbl_ovrd=off  reg_retiming=off  block_type=delay
      settings: block_version=11.4
  shift2 : xbsIndex_r4/Shift  shift_dir=Left  shift_bits=1  en=off  latency=0  precision=Full  arith_type="Signed  (2's comp)"  n_bits=16  bin_pt=14  quantization=Truncate  overflow=Wrap  dbl_ovrd=off  block_type=shift
  sync_delay : xbsIndex_r4/Delay  en=off  latency=1  dbl_ovrd=off  reg_retiming=off  block_type=delay
      settings: block_version=11.4
  out1 : Outport
  out2 : Outport  Port=2
  sync_out : Outport  Port=3
  wires:
  in/1 -> delay1/1, adder_tree2/1(sync), shift2/1, adder_tree2/2(din_1)  "adder_trees_out1"
  sync/1 -> sync_delay/1
  delay1/1 -> out1/1  "out1"
  shift2/1 -> adder_tree2/3(din_2)  "shift_out2"
  adder_tree2/2(dout) -> out2/1  "out2"
  sync_delay/1 -> sync_out/1

== system cic_filter_test_newnew_dec2_nonpoly_3/myCIC2/stage1/mult_cxi_blk4 ==
  in : Inport
  sync : Inport  Port=2
  adder_tree1 : Subsystem
  delay2 : xbsIndex_r4/Delay  en=off  latency=1  dbl_ovrd=off  reg_retiming=off  block_type=delay
      settings: block_version=11.4
  shift2 : xbsIndex_r4/Shift  shift_dir=Left  shift_bits=1  en=off  latency=0  precision=Full  arith_type="Signed  (2's comp)"  n_bits=16  bin_pt=14  quantization=Truncate  overflow=Wrap  dbl_ovrd=off  block_type=shift
  sync_delay : xbsIndex_r4/Delay  en=off  latency=1  dbl_ovrd=off  reg_retiming=off  block_type=delay
      settings: block_version=11.4
  out1 : Outport
  out2 : Outport  Port=2
  sync_out : Outport  Port=3
  wires:
  in/1 -> delay2/1, adder_tree1/1(sync), shift2/1, adder_tree1/2(din_1)  "adder_trees_out2"
  sync/1 -> sync_delay/1
  adder_tree1/2(dout) -> out1/1  "out1"
  shift2/1 -> adder_tree1/3(din_2)  "shift_out2"
  delay2/1 -> out2/1  "out2"
  sync_delay/1 -> sync_out/1

== system cic_filter_test_newnew_dec2_nonpoly_3/myCIC3/stage2/adder_tree2 ==
  sync : Inport
  din_1 : Inport  Port=2
  din_2 : Inport  Port=3
  din_3 : Inport  Port=4
  din_4 : Inport  Port=5
  adder_0 : xbsIndex_r4/AddSub  mode=Addition  use_carryin=off  use_carryout=off  en=off  latency=1  precision=Full  arith_type=Unsigned  n_bits=16  bin_pt=14  quantization="Round  (unbiased: +/- Inf)"  overflow=Saturate  dbl_ovrd=off  use_behavioral_HDL=on  hw_selection=Fabric  pipelined=off  block_type=addsub
  adder_1 : xbsIndex_r4/AddSub  mode=Addition  use_carryin=off  use_carryout=off  en=off  latency=1  precision=Full  arith_type=Unsigned  n_bits=16  bin_pt=14  quantization="Round  (unbiased: +/- Inf)"  overflow=Saturate  dbl_ovrd=off  use_behavioral_HDL=on  hw_selection=Fabric  pipelined=off  block_type=addsub
  adder_2 : xbsIndex_r4/AddSub  mode=Addition  use_carryin=off  use_carryout=off  en=off  latency=1  precision=Full  arith_type=Unsigned  n_bits=16  bin_pt=14  quantization="Round  (unbiased: +/- Inf)"  overflow=Saturate  dbl_ovrd=off  use_behavioral_HDL=on  hw_selection=Fabric  pipelined=off  block_type=addsub
  sync_delay : xbsIndex_r4/Delay  en=off  latency=2  dbl_ovrd=off  reg_retiming=off  block_type=delay
      settings: block_version=11.4
  zero_in : xbsIndex_r4/Constant  arith_type=Unsigned  const=0  n_bits=18  bin_pt=17  explicit_period=off  period=1  equ=P=C  opselect=C  inp2=PCIN>>17  opr=+  inp1=P  carry=CIN  dbl_ovrd=off  block_type=constant
      settings: block_version=11.4
  sync_out : Outport
  dout : Outport  Port=2
  wires:
  adder_0/1 -> adder_2/2
  din_4/1 -> adder_1/1
  din_1/1 -> adder_0/2
  sync_delay/1 -> sync_out/1
  sync/1 -> sync_delay/1
  din_2/1 -> adder_0/1
  din_3/1 -> adder_1/2
  adder_1/1 -> adder_2/1
  adder_2/1 -> dout/1

== system cic_filter_test_newnew_dec2_nonpoly_3/myCIC3/stage2/adder_tree4 ==
  sync : Inport
  din_1 : Inport  Port=2
  din_2 : Inport  Port=3
  din_3 : Inport  Port=4
  din_4 : Inport  Port=5
  adder_0 : xbsIndex_r4/AddSub  mode=Addition  use_carryin=off  use_carryout=off  en=off  latency=1  precision=Full  arith_type=Unsigned  n_bits=16  bin_pt=14  quantization="Round  (unbiased: +/- Inf)"  overflow=Saturate  dbl_ovrd=off  use_behavioral_HDL=on  hw_selection=Fabric  pipelined=off  block_type=addsub
  adder_1 : xbsIndex_r4/AddSub  mode=Addition  use_carryin=off  use_carryout=off  en=off  latency=1  precision=Full  arith_type=Unsigned  n_bits=16  bin_pt=14  quantization="Round  (unbiased: +/- Inf)"  overflow=Saturate  dbl_ovrd=off  use_behavioral_HDL=on  hw_selection=Fabric  pipelined=off  block_type=addsub
  adder_2 : xbsIndex_r4/AddSub  mode=Addition  use_carryin=off  use_carryout=off  en=off  latency=1  precision=Full  arith_type=Unsigned  n_bits=16  bin_pt=14  quantization="Round  (unbiased: +/- Inf)"  overflow=Saturate  dbl_ovrd=off  use_behavioral_HDL=on  hw_selection=Fabric  pipelined=off  block_type=addsub
  sync_delay : xbsIndex_r4/Delay  en=off  latency=2  dbl_ovrd=off  reg_retiming=off  block_type=delay
      settings: block_version=11.4
  zero_in : xbsIndex_r4/Constant  arith_type=Unsigned  const=0  n_bits=18  bin_pt=17  explicit_period=off  period=1  equ=P=C  opselect=C  inp2=PCIN>>17  opr=+  inp1=P  carry=CIN  dbl_ovrd=off  block_type=constant
      settings: block_version=11.4
  sync_out : Outport
  dout : Outport  Port=2
  wires:
  adder_0/1 -> adder_2/2
  din_4/1 -> adder_1/1
  din_1/1 -> adder_0/2
  sync_delay/1 -> sync_out/1
  sync/1 -> sync_delay/1
  din_2/1 -> adder_0/1
  din_3/1 -> adder_1/2
  adder_1/1 -> adder_2/1
  adder_2/1 -> dout/1

== system cic_filter_test_newnew_dec2_nonpoly_3/myCIC3/stage2_/adder_tree1 ==
  sync : Inport
  din_1 : Inport  Port=2
  din_2 : Inport  Port=3
  adder_0 : xbsIndex_r4/AddSub  mode=Addition  use_carryin=off  use_carryout=off  en=off  latency=1  precision=Full  arith_type=Unsigned  n_bits=16  bin_pt=14  quantization="Round  (unbiased: +/- Inf)"  overflow=Saturate  dbl_ovrd=off  use_behavioral_HDL=on  hw_selection=Fabric  pipelined=off  block_type=addsub
  sync_delay : xbsIndex_r4/Delay  en=off  latency=1  dbl_ovrd=off  reg_retiming=off  block_type=delay
      settings: block_version=11.4
  zero_in : xbsIndex_r4/Constant  arith_type=Unsigned  const=0  n_bits=18  bin_pt=17  explicit_period=off  period=1  equ=P=C  opselect=C  inp2=PCIN>>17  opr=+  inp1=P  carry=CIN  dbl_ovrd=off  block_type=constant
      settings: block_version=11.4
  sync_out : Outport
  dout : Outport  Port=2
  wires:
  din_1/1 -> adder_0/2
  sync_delay/1 -> sync_out/1
  sync/1 -> sync_delay/1
  din_2/1 -> adder_0/1
  adder_0/1 -> dout/1

== system cic_filter_test_newnew_dec2_nonpoly_3/myCIC3/stage2_/adder_tree2 ==
  sync : Inport
  din_1 : Inport  Port=2
  din_2 : Inport  Port=3
  adder_0 : xbsIndex_r4/AddSub  mode=Addition  use_carryin=off  use_carryout=off  en=off  latency=1  precision=Full  arith_type=Unsigned  n_bits=16  bin_pt=14  quantization="Round  (unbiased: +/- Inf)"  overflow=Saturate  dbl_ovrd=off  use_behavioral_HDL=on  hw_selection=Fabric  pipelined=off  block_type=addsub
  sync_delay : xbsIndex_r4/Delay  en=off  latency=1  dbl_ovrd=off  reg_retiming=off  block_type=delay
      settings: block_version=11.4
  zero_in : xbsIndex_r4/Constant  arith_type=Unsigned  const=0  n_bits=18  bin_pt=17  explicit_period=off  period=1  equ=P=C  opselect=C  inp2=PCIN>>17  opr=+  inp1=P  carry=CIN  dbl_ovrd=off  block_type=constant
      settings: block_version=11.4
  sync_out : Outport
  dout : Outport  Port=2
  wires:
  din_1/1 -> adder_0/2
  sync_delay/1 -> sync_out/1
  sync/1 -> sync_delay/1
  din_2/1 -> adder_0/1
  adder_0/1 -> dout/1

== system cic_filter_test_newnew_dec2_nonpoly_3/npcic nonpoly/stage1/polynomial ==
  in : Inport
  sync : Inport  Port=2
  adder_blk1 : xbsIndex_r4/AddSub  mode=Addition  use_carryin=off  use_carryout=off  en=off  latency=1  precision=Full  arith_type=Unsigned  n_bits=16  bin_pt=14  quantization=Truncate  overflow=Wrap  dbl_ovrd=off  use_behavioral_HDL=off  hw_selection=Fabric  pipelined=off  block_type=addsub
  adder_blk2 : xbsIndex_r4/AddSub  mode=Addition  use_carryin=off  use_carryout=off  en=off  latency=1  precision=Full  arith_type=Unsigned  n_bits=16  bin_pt=14  quantization=Truncate  overflow=Wrap  dbl_ovrd=off  use_behavioral_HDL=off  hw_selection=Fabric  pipelined=off  block_type=addsub
  adder_blk3 : xbsIndex_r4/AddSub  mode=Addition  use_carryin=off  use_carryout=off  en=off  latency=1  precision=Full  arith_type=Unsigned  n_bits=16  bin_pt=14  quantization=Truncate  overflow=Wrap  dbl_ovrd=off  use_behavioral_HDL=off  hw_selection=Fabric  pipelined=off  block_type=addsub
  delay0 : xbsIndex_r4/Delay  en=off  latency=1  dbl_ovrd=off  reg_retiming=off  block_type=delay
      settings: block_version=11.4
  shift_mult_array : Subsystem
  sync_delay1 : xbsIndex_r4/Delay  en=off  latency=1  dbl_ovrd=off  reg_retiming=off  block_type=delay
      settings: block_version=11.4
  out : Outport
  sync_out : Outport  Port=2
  wires:
  shift_mult_array/5(sync_out) -> sync_delay1/1  "sync_mult"
  adder_blk2/1 -> adder_blk3/1  "adder_ins3"
  shift_mult_array/3(out3) -> adder_blk2/2  "mult_out3"
  delay0/1 -> adder_blk1/1  "adder_ins1"
  shift_mult_array/1(out1) -> delay0/1  "mult_out1"
  sync/1 -> shift_mult_array/2(sync)
  in/1 -> shift_mult_array/1(in)
  shift_mult_array/2(out2) -> adder_blk1/2  "mult_out2"
  adder_blk1/1 -> adder_blk2/1  "adder_ins2"
  shift_mult_array/4(out4) -> adder_blk3/2  "mult_out4"
  adder_blk3/1 -> out/1  "adder_ins4"
  sync_delay1/1 -> sync_out/1

== system cic_filter_test_newnew_dec2_nonpoly_3/myCIC1/stage1/mult_cxi_blk1/adder_tree2 ==
  sync : Inport
  din_1 : Inport  Port=2
  din_2 : Inport  Port=3
  adder_0 : xbsIndex_r4/AddSub  mode=Addition  use_carryin=off  use_carryout=off  en=off  latency=1  precision=Full  arith_type=Unsigned  n_bits=16  bin_pt=14  quantization="Round  (unbiased: +/- Inf)"  overflow=Saturate  dbl_ovrd=off  use_behavioral_HDL=on  hw_selection=Fabric  pipelined=off  block_type=addsub
  sync_delay : xbsIndex_r4/Delay  en=off  latency=1  dbl_ovrd=off  reg_retiming=off  block_type=delay
      settings: block_version=11.4
  zero_in : xbsIndex_r4/Constant  arith_type=Unsigned  const=0  n_bits=18  bin_pt=17  explicit_period=off  period=1  equ=P=C  opselect=C  inp2=PCIN>>17  opr=+  inp1=P  carry=CIN  dbl_ovrd=off  block_type=constant
      settings: block_version=11.4
  sync_out : Outport
  dout : Outport  Port=2
  wires:
  din_1/1 -> adder_0/2
  sync_delay/1 -> sync_out/1
  sync/1 -> sync_delay/1
  din_2/1 -> adder_0/1
  adder_0/1 -> dout/1

== system cic_filter_test_newnew_dec2_nonpoly_3/myCIC1/stage1/mult_cxi_blk2/adder_tree1 ==
  sync : Inport
  din_1 : Inport  Port=2
  din_2 : Inport  Port=3
  adder_0 : xbsIndex_r4/AddSub  mode=Addition  use_carryin=off  use_carryout=off  en=off  latency=1  precision=Full  arith_type=Unsigned  n_bits=16  bin_pt=14  quantization="Round  (unbiased: +/- Inf)"  overflow=Saturate  dbl_ovrd=off  use_behavioral_HDL=on  hw_selection=Fabric  pipelined=off  block_type=addsub
  sync_delay : xbsIndex_r4/Delay  en=off  latency=1  dbl_ovrd=off  reg_retiming=off  block_type=delay
      settings: block_version=11.4
  zero_in : xbsIndex_r4/Constant  arith_type=Unsigned  const=0  n_bits=18  bin_pt=17  explicit_period=off  period=1  equ=P=C  opselect=C  inp2=PCIN>>17  opr=+  inp1=P  carry=CIN  dbl_ovrd=off  block_type=constant
      settings: block_version=11.4
  sync_out : Outport
  dout : Outport  Port=2
  wires:
  din_1/1 -> adder_0/2
  sync_delay/1 -> sync_out/1
  sync/1 -> sync_delay/1
  din_2/1 -> adder_0/1
  adder_0/1 -> dout/1

== system cic_filter_test_newnew_dec2_nonpoly_3/myCIC1/stage1/mult_cxi_blk3/adder_tree2 ==
  sync : Inport
  din_1 : Inport  Port=2
  din_2 : Inport  Port=3
  adder_0 : xbsIndex_r4/AddSub  mode=Addition  use_carryin=off  use_carryout=off  en=off  latency=1  precision=Full  arith_type=Unsigned  n_bits=16  bin_pt=14  quantization="Round  (unbiased: +/- Inf)"  overflow=Saturate  dbl_ovrd=off  use_behavioral_HDL=on  hw_selection=Fabric  pipelined=off  block_type=addsub
  sync_delay : xbsIndex_r4/Delay  en=off  latency=1  dbl_ovrd=off  reg_retiming=off  block_type=delay
      settings: block_version=11.4
  zero_in : xbsIndex_r4/Constant  arith_type=Unsigned  const=0  n_bits=18  bin_pt=17  explicit_period=off  period=1  equ=P=C  opselect=C  inp2=PCIN>>17  opr=+  inp1=P  carry=CIN  dbl_ovrd=off  block_type=constant
      settings: block_version=11.4
  sync_out : Outport
  dout : Outport  Port=2
  wires:
  din_1/1 -> adder_0/2
  sync_delay/1 -> sync_out/1
  sync/1 -> sync_delay/1
  din_2/1 -> adder_0/1
  adder_0/1 -> dout/1

== system cic_filter_test_newnew_dec2_nonpoly_3/myCIC1/stage1/mult_cxi_blk4/adder_tree1 ==
  sync : Inport
  din_1 : Inport  Port=2
  din_2 : Inport  Port=3
  adder_0 : xbsIndex_r4/AddSub  mode=Addition  use_carryin=off  use_carryout=off  en=off  latency=1  precision=Full  arith_type=Unsigned  n_bits=16  bin_pt=14  quantization="Round  (unbiased: +/- Inf)"  overflow=Saturate  dbl_ovrd=off  use_behavioral_HDL=on  hw_selection=Fabric  pipelined=off  block_type=addsub
  sync_delay : xbsIndex_r4/Delay  en=off  latency=1  dbl_ovrd=off  reg_retiming=off  block_type=delay
      settings: block_version=11.4
  zero_in : xbsIndex_r4/Constant  arith_type=Unsigned  const=0  n_bits=18  bin_pt=17  explicit_period=off  period=1  equ=P=C  opselect=C  inp2=PCIN>>17  opr=+  inp1=P  carry=CIN  dbl_ovrd=off  block_type=constant
      settings: block_version=11.4
  sync_out : Outport
  dout : Outport  Port=2
  wires:
  din_1/1 -> adder_0/2
  sync_delay/1 -> sync_out/1
  sync/1 -> sync_delay/1
  din_2/1 -> adder_0/1
  adder_0/1 -> dout/1

== system cic_filter_test_newnew_dec2_nonpoly_3/myCIC2/stage1/mult_cxi_blk1/adder_tree2 ==
  sync : Inport
  din_1 : Inport  Port=2
  din_2 : Inport  Port=3
  adder_0 : xbsIndex_r4/AddSub  mode=Addition  use_carryin=off  use_carryout=off  en=off  latency=1  precision=Full  arith_type=Unsigned  n_bits=16  bin_pt=14  quantization="Round  (unbiased: +/- Inf)"  overflow=Saturate  dbl_ovrd=off  use_behavioral_HDL=on  hw_selection=Fabric  pipelined=off  block_type=addsub
  sync_delay : xbsIndex_r4/Delay  en=off  latency=1  dbl_ovrd=off  reg_retiming=off  block_type=delay
      settings: block_version=11.4
  zero_in : xbsIndex_r4/Constant  arith_type=Unsigned  const=0  n_bits=18  bin_pt=17  explicit_period=off  period=1  equ=P=C  opselect=C  inp2=PCIN>>17  opr=+  inp1=P  carry=CIN  dbl_ovrd=off  block_type=constant
      settings: block_version=11.4
  sync_out : Outport
  dout : Outport  Port=2
  wires:
  din_1/1 -> adder_0/2
  sync_delay/1 -> sync_out/1
  sync/1 -> sync_delay/1
  din_2/1 -> adder_0/1
  adder_0/1 -> dout/1

== system cic_filter_test_newnew_dec2_nonpoly_3/myCIC2/stage1/mult_cxi_blk2/adder_tree1 ==
  sync : Inport
  din_1 : Inport  Port=2
  din_2 : Inport  Port=3
  adder_0 : xbsIndex_r4/AddSub  mode=Addition  use_carryin=off  use_carryout=off  en=off  latency=1  precision=Full  arith_type=Unsigned  n_bits=16  bin_pt=14  quantization="Round  (unbiased: +/- Inf)"  overflow=Saturate  dbl_ovrd=off  use_behavioral_HDL=on  hw_selection=Fabric  pipelined=off  block_type=addsub
  sync_delay : xbsIndex_r4/Delay  en=off  latency=1  dbl_ovrd=off  reg_retiming=off  block_type=delay
      settings: block_version=11.4
  zero_in : xbsIndex_r4/Constant  arith_type=Unsigned  const=0  n_bits=18  bin_pt=17  explicit_period=off  period=1  equ=P=C  opselect=C  inp2=PCIN>>17  opr=+  inp1=P  carry=CIN  dbl_ovrd=off  block_type=constant
      settings: block_version=11.4
  sync_out : Outport
  dout : Outport  Port=2
  wires:
  din_1/1 -> adder_0/2
  sync_delay/1 -> sync_out/1
  sync/1 -> sync_delay/1
  din_2/1 -> adder_0/1
  adder_0/1 -> dout/1

== system cic_filter_test_newnew_dec2_nonpoly_3/myCIC2/stage1/mult_cxi_blk3/adder_tree2 ==
  sync : Inport
  din_1 : Inport  Port=2
  din_2 : Inport  Port=3
  adder_0 : xbsIndex_r4/AddSub  mode=Addition  use_carryin=off  use_carryout=off  en=off  latency=1  precision=Full  arith_type=Unsigned  n_bits=16  bin_pt=14  quantization="Round  (unbiased: +/- Inf)"  overflow=Saturate  dbl_ovrd=off  use_behavioral_HDL=on  hw_selection=Fabric  pipelined=off  block_type=addsub
  sync_delay : xbsIndex_r4/Delay  en=off  latency=1  dbl_ovrd=off  reg_retiming=off  block_type=delay
      settings: block_version=11.4
  zero_in : xbsIndex_r4/Constant  arith_type=Unsigned  const=0  n_bits=18  bin_pt=17  explicit_period=off  period=1  equ=P=C  opselect=C  inp2=PCIN>>17  opr=+  inp1=P  carry=CIN  dbl_ovrd=off  block_type=constant
      settings: block_version=11.4
  sync_out : Outport
  dout : Outport  Port=2
  wires:
  din_1/1 -> adder_0/2
  sync_delay/1 -> sync_out/1
  sync/1 -> sync_delay/1
  din_2/1 -> adder_0/1
  adder_0/1 -> dout/1

== system cic_filter_test_newnew_dec2_nonpoly_3/myCIC2/stage1/mult_cxi_blk4/adder_tree1 ==
  sync : Inport
  din_1 : Inport  Port=2
  din_2 : Inport  Port=3
  adder_0 : xbsIndex_r4/AddSub  mode=Addition  use_carryin=off  use_carryout=off  en=off  latency=1  precision=Full  arith_type=Unsigned  n_bits=16  bin_pt=14  quantization="Round  (unbiased: +/- Inf)"  overflow=Saturate  dbl_ovrd=off  use_behavioral_HDL=on  hw_selection=Fabric  pipelined=off  block_type=addsub
  sync_delay : xbsIndex_r4/Delay  en=off  latency=1  dbl_ovrd=off  reg_retiming=off  block_type=delay
      settings: block_version=11.4
  zero_in : xbsIndex_r4/Constant  arith_type=Unsigned  const=0  n_bits=18  bin_pt=17  explicit_period=off  period=1  equ=P=C  opselect=C  inp2=PCIN>>17  opr=+  inp1=P  carry=CIN  dbl_ovrd=off  block_type=constant
      settings: block_version=11.4
  sync_out : Outport
  dout : Outport  Port=2
  wires:
  din_1/1 -> adder_0/2
  sync_delay/1 -> sync_out/1
  sync/1 -> sync_delay/1
  din_2/1 -> adder_0/1
  adder_0/1 -> dout/1

== system cic_filter_test_newnew_dec2_nonpoly_3/npcic nonpoly/stage1/polynomial/shift_mult_array ==
  in : Inport
  sync : Inport  Port=2
  adder_tree2 : Subsystem
  delay1 : xbsIndex_r4/Delay  en=off  latency=1  dbl_ovrd=off  reg_retiming=off  block_type=delay
      settings: block_version=11.4
  shift2 : xbsIndex_r4/Shift  shift_dir=Left  shift_bits=1  en=off  latency=0  precision=User Defined  arith_type="Signed  (2's comp)"  n_bits=9  bin_pt=3  quantization=Truncate  overflow=Wrap  dbl_ovrd=off  block_type=shift
  sync_delay : xbsIndex_r4/Delay  en=off  latency=1  dbl_ovrd=off  reg_retiming=off  block_type=delay
      settings: block_version=11.4
  out1 : Outport
  out2 : Outport  Port=2
  out3 : Outport  Port=3
  out4 : Outport  Port=4
  sync_out : Outport  Port=5
  wires:
  in/1 -> delay1/1, adder_tree2/1(sync), shift2/1, adder_tree2/2(din_1)  "adder_trees_out1"
  adder_tree2/2(dout) -> out3/1, out2/1  "out2"
  delay1/1 -> out1/1, out4/1  "out1"
  sync/1 -> sync_delay/1
  shift2/1 -> adder_tree2/3(din_2)  "shift_out2"
  sync_delay/1 -> sync_out/1

== system cic_filter_test_newnew_dec2_nonpoly_3/npcic nonpoly/stage1/polynomial/shift_mult_array/adder_tree2 ==
  sync : Inport
  din_1 : Inport  Port=2
  din_2 : Inport  Port=3
  adder_0 : xbsIndex_r4/AddSub  mode=Addition  use_carryin=off  use_carryout=off  en=off  latency=1  precision=Full  arith_type=Unsigned  n_bits=16  bin_pt=14  quantization="Round  (unbiased: +/- Inf)"  overflow=Saturate  dbl_ovrd=off  use_behavioral_HDL=on  hw_selection=Fabric  pipelined=off  block_type=addsub
  sync_delay : xbsIndex_r4/Delay  en=off  latency=1  dbl_ovrd=off  reg_retiming=off  block_type=delay
      settings: block_version=11.4
  zero_in : xbsIndex_r4/Constant  arith_type=Unsigned  const=0  n_bits=18  bin_pt=17  explicit_period=off  period=1  equ=P=C  opselect=C  inp2=PCIN>>17  opr=+  inp1=P  carry=CIN  dbl_ovrd=off  block_type=constant
      settings: block_version=11.4
  sync_out : Outport
  dout : Outport  Port=2
  wires:
  din_1/1 -> adder_0/2
  sync_delay/1 -> sync_out/1
  sync/1 -> sync_delay/1
  din_2/1 -> adder_0/1
  adder_0/1 -> dout/1
